simulink model "MSX60_signle_cell"  (Simulink 7.9)
settings: Solver=ode14x  StartTime=0.0  StopTime=220  FixedStep=0.05  RelTol=1e-4
values from neighbouring files (symbols this model uses):
  n = 1.3    [MSX60DS.m]    (also in MSX60_10_RL.m; MSX60_10_by2_with_PandO.m; MSX60_10_by2_with_PandO_PS.m; MSX60_10_by2_with_PandO_US (1).m)
  Ns = 1    [MSX60DS.m]    (also in MSX60_10_RL.m; MSX60_10_by2_with_PandO.m; MSX60_10_by2_with_PandO_PS.m; MSX60_10_by2_with_PandO_US (1).m)
  Rs = 0.58    [MSX60DS.m]    (also in MSX60_10_RL.m; MSX60_10_by2_with_PandO.m; MSX60_10_by2_with_PandO_PS.m; MSX60_10_by2_with_PandO_US (1).m)
  Voc = Voc(1)    [MSX60DS.m]    (also in MSX60_10_RL.m = 21.1; MSX60_10_by2_with_PandO.m = 21.1; MSX60_10_by2_with_PandO_PS.m = 21.1; MSX60_10_by2_with_PandO_US (1).m = 21.1)
libraries: fl_lib x4, nesl_utility x3, elec_lib x1, simulink x1
settings Model: Creator=pc1  LastModifiedBy=pc1
settings SolverCC: SolverJacobianMethodControl=SparsePerturbation
settings DataIOCC: SaveState=on

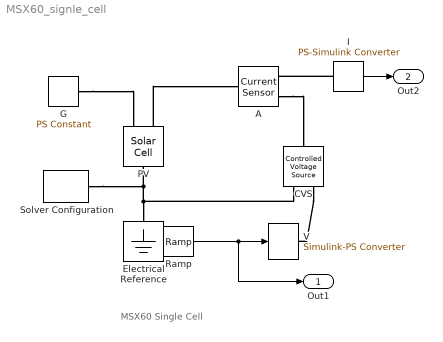
== system MSX60_signle_cell ==
  note: MSX60 Single Cell
  A : fl_lib/Electrical/Electrical Sensors/Current Sensor  i1_Log=off  v1_Log=off  LocalVarNames=|i1|v1  LocalVarDescs=|i1|v1  LocalVarLogging=[0 0]
  CVS : fl_lib/Electrical/Electrical Sources/Controlled Voltage Source  i_Log=off  v_Log=off  LocalVarNames=|i|v  LocalVarDescs=|i|v  LocalVarLogging=[0 0]
  Electrical Reference : fl_lib/Electrical/Electrical Elements/Electrical Reference  i_Log=off  LocalVarNames=|i  LocalVarDescs=|i  LocalVarLogging=0
  G : fl_lib/Physical Signals/Sources/PS Constant  constant=G  LocalVarLogging=[]
  I : nesl_utility/PS-Simulink Converter  PhysicalDomain=network_engine_domain  LeftPortType=input  RightPortType=output  SubClassName=ps_output  Unit=1  AffineConversion=off
  PV : elec_lib/Sources/Solar Cell  prm=1  Isc=Isc A  Voc=Voc*Ns V  Is=1e-6 A  Is2=0 A  Iph=3.8 A  Ir0=Gstc W/m^2  ec=n*Voc*Ns  N2=0  Rs=Rs*Ns Ohm  Rp=Inf Ohm  TIPH1=0 1/K  EG=1.11 eV  TXIS1=3  TXIS2=3  TRS1=0  TRP1=0  Tmeas=25 C  TFIXED=25 C  LocalVarLogging=[]  thermal_mass=100 J/K  initial_temperature=25 C
  Ramp : simulink/Sources/Ramp  slope=1  start=1  X0=0
  Solver Configuration : nesl_utility/Solver Configuration  PhysicalDomain=network_engine_domain  LeftPortType=input  RightPortType=generic  SubClassName=solver  UseCustomDae=off  DoDC=on  ResidualTolerance=1e-9  UseLocalSolver=off  LocalSolverChoice=NE_BACKWARD_EULER_ADVANCER  LocalSolverSampleTime=.001  DoFixedCost=off  MaxNonlinIter=3  MaxModeIter=2  LinearAlgebra=Sparse  Accelerate=off  Profile=off  UseLocalSampling=off  DelaysMemoryBudget=1024
  V : nesl_utility/Simulink-PS Converter  PhysicalDomain=network_engine_domain  LeftPortType=input  RightPortType=output  SubClassName=ps_input  Unit=1  AffineConversion=off  InputFilterTimeConstant=.001  UdotUserProvided=[]  SimscapeFilterOrder=1  InputFiltering=off
  Out1 : Outport
  Out2 : Outport  Port=2
  wires:
  Ramp/1 -> V/1, Out1/1
  I/1 -> Out2/1
  connections:
  CVS/RConn2 -- Solver Configuration/RConn1 -- PV/RConn1 -- Electrical Reference/LConn1
  A/RConn2 -- CVS/LConn1
  CVS/RConn1 -- V/RConn1
  I/LConn1 -- A/RConn1
  PV/LConn2 -- A/LConn1
  G/RConn1 -- PV/LConn1
